simulink model "sampleModel9_EMI_Var"  (R2017a)
settings: Solver=VariableStepAuto  StartTime=0.0  StopTime=10.0  RelTol=1e-3
undefined symbols (not defined in the file or in its folder): DiscIntNeverNeededParam
libraries: simulink x42
settings Model: Creator=cyfuzz  LastModifiedBy=cyfuzz

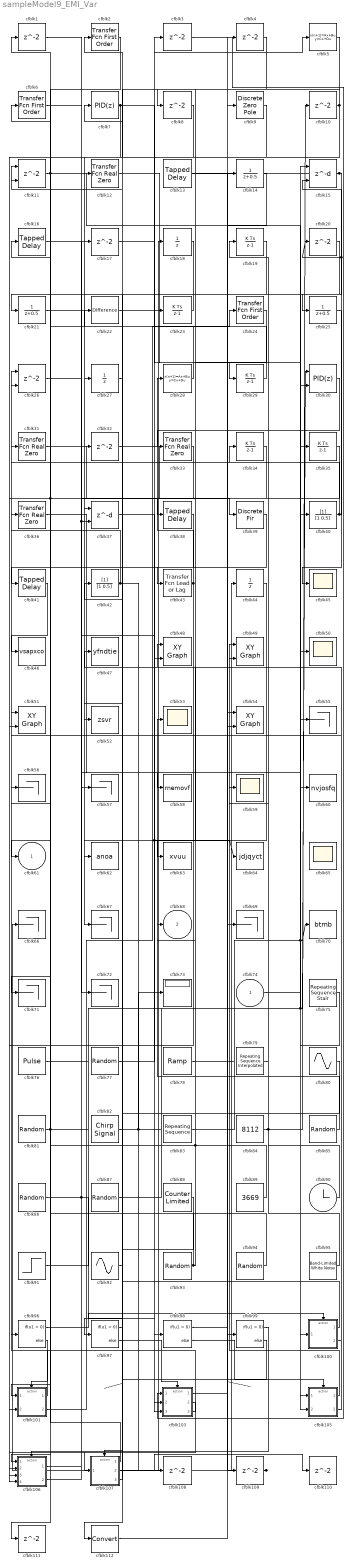
== system sampleModel9_EMI_Var ==
  cfblk74 : Inport
  cfblk{1,3..4,8,10,17,20,32,108..111} (12 alike) : Delay  SampleTime=1
  cfblk100 : Subsystem  TreatAsAtomicUnit=on
  cfblk101 : Subsystem  TreatAsAtomicUnit=on
  cfblk103 : Subsystem  TreatAsAtomicUnit=on
  cfblk105 : Subsystem  TreatAsAtomicUnit=on
  cfblk106 : Subsystem  TreatAsAtomicUnit=on
  cfblk107 : Subsystem  TreatAsAtomicUnit=on
  cfblk11 : Delay  ShowEnablePort=on  SampleTime=1
      settings: InputPortMap=u0,e6
  cfblk112 : DataTypeConversion
  cfblk{12,31,33,36} (4 alike) : simulink/Discrete/Transfer Fcn Real Zero  ZeroZ=0.75  ICPrevInput=0.0  DoSatur=off
      settings: SourceProductName=Simulink  SourceProductBaseCode=SL
  cfblk{13,16,38,41} (4 alike) : simulink/Discrete/Tapped Delay  vinit=0.0  samptime=-1  NumDelays=1  DelayOrder=Oldest  includeCurrent=off
  cfblk14 : DiscreteTransferFcn  SampleTime=1
  cfblk15 : Delay  DelayLengthSource=Input port  SampleTime=1
      settings: InputPortMap=u0,p1
  cfblk18 : UnitDelay
  cfblk{19,23,29,34..35} (5 alike) : DiscreteIntegrator  InitialConditionSetting=State (most efficient)  ICPrevOutput=DiscIntNeverNeededParam  ICPrevScaledInput=DiscIntNeverNeededParam
  cfblk2 : simulink/Discrete/Transfer Fcn First Order  PoleZ=0.95  ICPrevOutput=0.0  DoSatur=off
      settings: SourceProductName=Simulink
  cfblk21 : DiscreteTransferFcn  SampleTime=1
  cfblk22 : simulink/Discrete/Difference  ICPrevInput=0.0  OutMin=[]  OutMax=[]  OutDataTypeStr=Inherit: Inherit via back propagation  OutDataType=fixdt(1, 16)  OutScaling=2^-10  DoSatur=off
  cfblk24 : simulink/Discrete/Transfer Fcn First Order  PoleZ=0.95  ICPrevOutput=0.0  DoSatur=off
      settings: SourceProductName=Simulink
  cfblk25 : DiscreteTransferFcn  SampleTime=1
  cfblk26 : Delay  ShowEnablePort=on  SampleTime=1
      settings: InputPortMap=u0,e6
  cfblk27 : UnitDelay
  cfblk28 : DiscreteStateSpace
  cfblk30 : simulink/Continuous/PID Controller (2DOF)  Controller=PID  TimeDomain=Discrete-time  SampleTime=1  IntegratorMethod=Forward Euler  FilterMethod=Forward Euler  Form=Parallel  UseFilter=on  ControllerParametersSource=internal  P=1  I=1  D=0  N=100  b=1  c=1  InitialConditionSource=internal  InitialConditionForIntegrator=0  InitialConditionForFilter=0  ExternalReset=none  LimitOutput=off  UpperSaturationLimit=inf  LowerSaturationLimit=-inf  LinearizeAsGain=off  AntiWindupMode=none  Kb=1  TrackingMode=off  Kt=1  PParamMin=[]  PParamMax=[]  IParamMin=[]  IParamMax=[]  DParamMin=[]  DParamMax=[]  NParamMin=[]  NParamMax=[]  bParamMin=[]  bParamMax=[]  cParamMin=[]  cParamMax=[]  KbParamMin=[]  KbParamMax=[]  KtParamMin=[]  KtParamMax=[]  POutMin=[]  POutMax=[]  IOutMin=[]  IOutMax=[]  DOutMin=[]  DOutMax=[]  NOutMin=[]  NOutMax=[]  bOutMin=[]  bOutMax=[]  cOutMin=[]  cOutMax=[]  KbOutMin=[]  KbOutMax=[]  KtOutMin=[]  KtOutMax=[]  IntegratorOutMin=[]  IntegratorOutMax=[]  FilterOutMin=[]  FilterOutMax=[]  SumOutMin=[]  SumOutMax=[]  Sum1OutMin=[]  Sum1OutMax=[]  Sum2OutMin=[]  Sum2OutMax=[]  Sum3OutMin=[]  Sum3OutMax=[]  SumI1OutMin=[]  SumI1OutMax=[]  SumI2OutMin=[]  SumI2OutMax=[]  SumI3OutMin=[]  SumI3OutMax=[]  SumDOutMin=[]  SumDOutMax=[]  SaturationOutMin=[]  SaturationOutMax=[]  IntegratorContinuousStateAttributes=''  IntegratorStateMustResolveToSignalObject=off  IntegratorRTWStateStorageClass=Auto  FilterContinuousStateAttributes=''  FilterStateMustResolveToSignalObject=off  FilterRTWStateStorageClass=Auto  DifferentiatorICPrevScaledInput=0  DifferentiatorOutMin=[]  DifferentiatorOutMax=[]  InitialConditionSetting=State (most efficient)
  cfblk37 : Delay  DelayLengthSource=Input port  SampleTime=1
      settings: InputPortMap=u0,p1
  cfblk39 : DiscreteFir  SampleTime=1
  cfblk40 : DiscreteFilter  SampleTime=1
  cfblk42 : DiscreteFilter  SampleTime=1
  cfblk43 : simulink/Discrete/Transfer Fcn Lead or Lag  PoleZ=0.95  ZeroZ=0.75  ICPrevOutput=0.0  ICPrevInput=0.0  DoSatur=off
      settings: SourceProductName=Simulink  SourceProductBaseCode=SL
  cfblk44 : UnitDelay
  cfblk{45,50,53,59,65} (5 alike) : Scope
      cfblk65 settings: Floating=on
  cfblk46 : ToWorkspace  VariableName=vsapxco  SaveFormat=Timeseries  SampleTime=-1
  cfblk47 : ToWorkspace  VariableName=yfndtie  SaveFormat=Timeseries  SampleTime=-1
  cfblk{48..49,51,54} (4 alike) : simulink/Sinks/XY Graph  xmin=-1  xmax=1  ymin=-1  ymax=1  st=-1
  cfblk5 : DiscreteStateSpace
  cfblk52 : ToFile  Filename=zsvr  SaveFormat=Timeseries
  cfblk{55..57,66..67,69,71..72} (8 alike) : Terminator
  cfblk58 : ToWorkspace  VariableName=rnemovf  SaveFormat=Timeseries  SampleTime=-1
  cfblk6 : simulink/Discrete/Transfer Fcn First Order  PoleZ=0.95  ICPrevOutput=0.0  DoSatur=off
      settings: SourceProductName=Simulink
  cfblk60 : ToWorkspace  VariableName=nvjosfq  SaveFormat=Timeseries  SampleTime=-1
  cfblk62 : ToFile  Filename=anoa  SaveFormat=Timeseries
  cfblk63 : ToFile  Filename=xvuu  SaveFormat=Timeseries
  cfblk64 : ToWorkspace  VariableName=jdjqyct  SaveFormat=Timeseries  SampleTime=-1
  cfblk7 : simulink/Continuous/PID Controller  Controller=PID  TimeDomain=Discrete-time  SampleTime=1  IntegratorMethod=Forward Euler  FilterMethod=Forward Euler  Form=Parallel  UseFilter=on  ControllerParametersSource=internal  P=1  I=1  D=0  N=100  InitialConditionSource=internal  InitialConditionForIntegrator=0  InitialConditionForFilter=0  ExternalReset=none  LimitOutput=off  UpperSaturationLimit=inf  LowerSaturationLimit=-inf  LinearizeAsGain=off  AntiWindupMode=none  Kb=1  TrackingMode=off  Kt=1  PParamMin=[]  PParamMax=[]  IParamMin=[]  IParamMax=[]  DParamMin=[]  DParamMax=[]  NParamMin=[]  NParamMax=[]  KbParamMin=[]  KbParamMax=[]  KtParamMin=[]  KtParamMax=[]  POutMin=[]  POutMax=[]  IOutMin=[]  IOutMax=[]  DOutMin=[]  DOutMax=[]  NOutMin=[]  NOutMax=[]  KbOutMin=[]  KbOutMax=[]  KtOutMin=[]  KtOutMax=[]  IntegratorOutMin=[]  IntegratorOutMax=[]  FilterOutMin=[]  FilterOutMax=[]  SumOutMin=[]  SumOutMax=[]  SumI1OutMin=[]  SumI1OutMax=[]  SumI2OutMin=[]  SumI2OutMax=[]  SumI3OutMin=[]  SumI3OutMax=[]  SumDOutMin=[]  SumDOutMax=[]  SaturationOutMin=[]  SaturationOutMax=[]  IntegratorContinuousStateAttributes=''  IntegratorStateMustResolveToSignalObject=off  IntegratorRTWStateStorageClass=Auto  FilterContinuousStateAttributes=''  FilterStateMustResolveToSignalObject=off  FilterRTWStateStorageClass=Auto  DifferentiatorICPrevScaledInput=0  DifferentiatorOutMin=[]  DifferentiatorOutMax=[]  InitialConditionSetting=State (most efficient)
  cfblk70 : ToFile  Filename=btmb  SaveFormat=Timeseries
  cfblk73 : Display
  cfblk75 : simulink/Sources/Repeating Sequence Stair  OutValues=[3 1 4 2 1].'  tsamp=-1  OutMin=[]  OutMax=[]  OutDataTypeStr=double  OutputDataTypeScalingMode=double  OutDataType=fixdt(0,8)  ConRadixGroup=Best Precision: Vector-wise  OutScaling=2^-12
  cfblk76 : DiscretePulseGenerator  PulseType=Time based  Period=10  PulseWidth=5
  cfblk{77,81,85..87,93..94} (7 alike) : RandomNumber  SampleTime=0.1
  cfblk78 : simulink/Sources/Ramp  slope=1  start=0  X0=0
  cfblk79 : simulink/Sources/Repeating Sequence Interpolated  OutValues=[3 1 4 2 1].'  TimeValues=[0 0.1 0.5 0.6 1].'  LookUpMeth=Interpolation-Use End Values  tsamp=0.01  OutMin=[]  OutMax=[]  OutDataTypeStr=double  OutputDataTypeScalingMode=double  OutDataType=fixdt(0,8)  OutScaling=2^-10
  cfblk80 : Sin  SampleTime=0
  cfblk82 : simulink/Sources/Chirp Signal  f1=0.1  T=100  f2=1
  cfblk83 : simulink/Sources/Repeating Sequence  rep_seq_t=[0 2]  rep_seq_y=[0 2]
  cfblk84 : Constant  Value=8112
  cfblk88 : simulink/Sources/Counter Limited  uplimit=7  tsamp=-1
  cfblk89 : Constant  Value=3669
  cfblk9 : DiscreteZeroPole  Poles=[0 0.5]  Gain=1
  cfblk90 : Clock
  cfblk91 : Step  After=97  SampleTime=0
  cfblk92 : Sin  SampleTime=0
  cfblk95 : simulink/Sources/Band-Limited White Noise  Cov=[0.1]  Ts=0.1  seed=[23341]
  cfblk{96..99} (4 alike) : If  SampleTime=1
  cfblk61 : Outport
  cfblk68 : Outport  Port=2
  wires:
  cfblk85/1 -> cfblk53/1
  cfblk101/1(cfblk2) -> cfblk26/1
  cfblk8/1 -> cfblk67/1
  cfblk101/2(cfblk13) -> cfblk24/1
  cfblk84/1 -> cfblk10/1, cfblk59/1
  cfblk86/1 -> cfblk57/1, cfblk103/3(cfblk7)
  cfblk92/1 -> cfblk2/1
  cfblk9/1 -> cfblk41/1
  cfblk10/1 -> cfblk8/1, cfblk33/1
  cfblk106/1(cfblk2) -> cfblk17/1
  cfblk43/1 -> cfblk28/1, cfblk106/4(cfblk8)
  cfblk20/1 -> cfblk97/1
  cfblk30/1 -> cfblk63/1
  cfblk76/1 -> cfblk30/1, cfblk30/2
  cfblk11/1 -> cfblk35/1, cfblk111/1
  cfblk38/1 -> cfblk106/1(cfblk1)
  cfblk25/1 -> cfblk45/1
  cfblk95/1 -> cfblk19/1
  cfblk40/1 -> cfblk15/2, cfblk20/1, cfblk26/2
  cfblk105/1(cfblk2) -> cfblk49/1
  cfblk21/1 -> cfblk27/1
  cfblk42/1 -> cfblk31/1, cfblk108/1
  cfblk18/1 -> cfblk37/1
  cfblk22/1 -> cfblk60/1
  cfblk36/1 -> cfblk105/1(cfblk1)
  cfblk74/1 -> cfblk40/1
  cfblk91/1 -> cfblk55/1
  cfblk12/1 -> cfblk100/1(cfblk1)
  cfblk27/1 -> cfblk7/1
  cfblk31/1 -> cfblk54/1
  cfblk3/1 -> cfblk103/1(cfblk1)
  cfblk80/1 -> cfblk107/1(cfblk1)
  cfblk14/1 -> cfblk54/2
  cfblk77/1 -> cfblk3/1
  cfblk87/1 -> cfblk4/1
  cfblk23/1 -> cfblk21/1
  cfblk15/1 -> cfblk25/1, cfblk13/1
  cfblk2/1 -> cfblk71/1
  cfblk106/2(cfblk9) -> cfblk32/1
  cfblk7/1 -> cfblk29/1, cfblk101/2(cfblk12)
  cfblk81/1 -> cfblk56/1, cfblk23/1
  cfblk103/1(cfblk2) -> cfblk99/1
  cfblk93/1 -> cfblk6/1, cfblk48/1
  cfblk37/1 -> cfblk98/1, cfblk64/1
  cfblk5/1 -> cfblk12/1
  cfblk94/1 -> cfblk22/1
  cfblk100/1(cfblk2) -> cfblk42/1
  cfblk89/1 -> cfblk16/1, cfblk68/1
  cfblk105/2(cfblk13) -> cfblk51/1
  cfblk4/1 -> cfblk43/1
  cfblk75/1 -> cfblk105/2(cfblk12)
  cfblk41/1 -> cfblk46/1
  cfblk24/1 -> cfblk38/1
  cfblk17/1 -> cfblk5/1
  cfblk79/1 -> cfblk49/2
  cfblk100/2(cfblk10) -> cfblk47/1
  cfblk16/1 -> cfblk72/1
  cfblk78/1 -> cfblk15/1
  cfblk6/1 -> cfblk39/1
  cfblk44/1 -> cfblk62/1
  cfblk39/1 -> cfblk103/2(cfblk6)
  cfblk35/1 -> cfblk52/1
  cfblk34/1 -> cfblk106/2(cfblk6)
  cfblk107/1(cfblk2) -> cfblk36/1
  cfblk103/2(cfblk8) -> cfblk106/3(cfblk7)
  cfblk83/1 -> cfblk70/1, cfblk50/1
  cfblk32/1 -> cfblk69/1
  cfblk26/1 -> cfblk37/2, cfblk48/2
  cfblk19/1 -> cfblk101/1(cfblk1)
  cfblk28/1 -> cfblk11/1
  cfblk1/1 -> cfblk58/1
  cfblk29/1 -> cfblk1/1
  cfblk33/1 -> cfblk61/1, cfblk51/2
  cfblk82/1 -> cfblk14/1, cfblk73/1
  cfblk90/1 -> cfblk34/1
  cfblk103/3(cfblk9) -> cfblk96/1
  cfblk107/3(cfblk7) -> cfblk11/2
  cfblk96/1 -> cfblk100/Action
  cfblk96/2 -> cfblk101/Action
  cfblk97/1 -> ?
  cfblk97/2 -> cfblk103/Action
  cfblk98/1 -> ?
  cfblk98/2 -> cfblk105/Action
  cfblk99/1 -> cfblk106/Action
  cfblk99/2 -> cfblk107/Action
  cfblk13/1 -> cfblk109/1
  cfblk107/2(cfblk6) -> cfblk110/1
  cfblk88/1 -> cfblk112/1
  cfblk112/1 -> cfblk9/1
  cfblk109/1 -> cfblk18/1, cfblk44/1, cfblk66/1

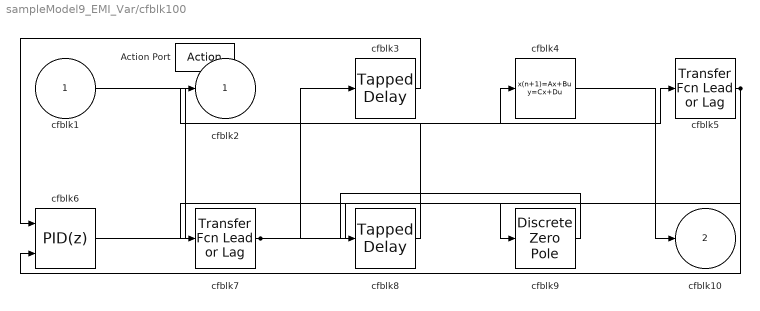
== system sampleModel9_EMI_Var/cfblk100 ==
  cfblk1 : Inport
  Action Port : ActionPort  ActionType=then
  cfblk3 : simulink/Discrete/Tapped Delay  vinit=0.0  samptime=-1  NumDelays=1  DelayOrder=Oldest  includeCurrent=off
  cfblk4 : DiscreteStateSpace  SampleTime=-1
  cfblk5 : simulink/Discrete/Transfer Fcn Lead or Lag  PoleZ=0.95  ZeroZ=0.75  ICPrevOutput=0.0  ICPrevInput=0.0  DoSatur=off
      settings: SourceProductName=Simulink  SourceProductBaseCode=SL
  cfblk6 : simulink/Continuous/PID Controller (2DOF)  Controller=PID  TimeDomain=Discrete-time  SampleTime=-1  IntegratorMethod=Forward Euler  FilterMethod=Forward Euler  Form=Parallel  UseFilter=on  ControllerParametersSource=internal  P=1  I=1  D=0  N=100  b=1  c=1  InitialConditionSource=internal  InitialConditionForIntegrator=0  InitialConditionForFilter=0  ExternalReset=none  LimitOutput=off  UpperSaturationLimit=inf  LowerSaturationLimit=-inf  LinearizeAsGain=off  AntiWindupMode=none  Kb=1  TrackingMode=off  Kt=1  PParamMin=[]  PParamMax=[]  IParamMin=[]  IParamMax=[]  DParamMin=[]  DParamMax=[]  NParamMin=[]  NParamMax=[]  bParamMin=[]  bParamMax=[]  cParamMin=[]  cParamMax=[]  KbParamMin=[]  KbParamMax=[]  KtParamMin=[]  KtParamMax=[]  POutMin=[]  POutMax=[]  IOutMin=[]  IOutMax=[]  DOutMin=[]  DOutMax=[]  NOutMin=[]  NOutMax=[]  bOutMin=[]  bOutMax=[]  cOutMin=[]  cOutMax=[]  KbOutMin=[]  KbOutMax=[]  KtOutMin=[]  KtOutMax=[]  IntegratorOutMin=[]  IntegratorOutMax=[]  FilterOutMin=[]  FilterOutMax=[]  SumOutMin=[]  SumOutMax=[]  Sum1OutMin=[]  Sum1OutMax=[]  Sum2OutMin=[]  Sum2OutMax=[]  Sum3OutMin=[]  Sum3OutMax=[]  SumI1OutMin=[]  SumI1OutMax=[]  SumI2OutMin=[]  SumI2OutMax=[]  SumI3OutMin=[]  SumI3OutMax=[]  SumDOutMin=[]  SumDOutMax=[]  SaturationOutMin=[]  SaturationOutMax=[]  IntegratorContinuousStateAttributes=''  IntegratorStateMustResolveToSignalObject=off  IntegratorRTWStateStorageClass=Auto  FilterContinuousStateAttributes=''  FilterStateMustResolveToSignalObject=off  FilterRTWStateStorageClass=Auto  DifferentiatorICPrevScaledInput=0  DifferentiatorOutMin=[]  DifferentiatorOutMax=[]  InitialConditionSetting=State (most efficient)
  cfblk7 : simulink/Discrete/Transfer Fcn Lead or Lag  PoleZ=0.95  ZeroZ=0.75  ICPrevOutput=0.0  ICPrevInput=0.0  DoSatur=off
      settings: SourceProductName=Simulink  SourceProductBaseCode=SL
  cfblk8 : simulink/Discrete/Tapped Delay  vinit=0.0  samptime=-1  NumDelays=1  DelayOrder=Oldest  includeCurrent=off
  cfblk9 : DiscreteZeroPole  Poles=[0 0.5]  Gain=1  SampleTime=-1
  cfblk2 : Outport
  cfblk10 : Outport  Port=2
  wires:
  cfblk1/1 -> cfblk5/1
  cfblk6/1 -> cfblk4/1
  cfblk3/1 -> cfblk6/1
  cfblk5/1 -> cfblk6/2, cfblk7/1
  cfblk7/1 -> cfblk9/1, cfblk3/1
  cfblk4/1 -> cfblk10/1
  cfblk9/1 -> cfblk8/1
  cfblk8/1 -> cfblk2/1

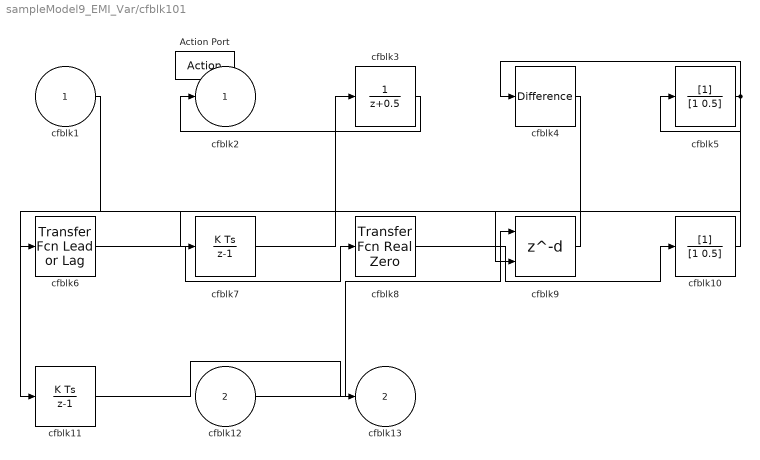
== system sampleModel9_EMI_Var/cfblk101 ==
  cfblk1 : Inport
  cfblk12 : Inport  Port=2
  Action Port : ActionPort  ActionType=else
  cfblk10 : DiscreteFilter
  cfblk11 : DiscreteIntegrator  InitialConditionSetting=State (most efficient)  SampleTime=-1  ICPrevOutput=DiscIntNeverNeededParam  ICPrevScaledInput=DiscIntNeverNeededParam
  cfblk3 : DiscreteTransferFcn
  cfblk4 : simulink/Discrete/Difference  ICPrevInput=0.0  OutMin=[]  OutMax=[]  OutDataTypeStr=Inherit: Inherit via back propagation  OutDataType=fixdt(1, 16)  OutScaling=2^-10  DoSatur=off
  cfblk5 : DiscreteFilter
  cfblk6 : simulink/Discrete/Transfer Fcn Lead or Lag  PoleZ=0.95  ZeroZ=0.75  ICPrevOutput=0.0  ICPrevInput=0.0  DoSatur=off
      settings: SourceProductName=Simulink  SourceProductBaseCode=SL
  cfblk7 : DiscreteIntegrator  InitialConditionSetting=State (most efficient)  SampleTime=-1  ICPrevOutput=DiscIntNeverNeededParam  ICPrevScaledInput=DiscIntNeverNeededParam
  cfblk8 : simulink/Discrete/Transfer Fcn Real Zero  ZeroZ=0.75  ICPrevInput=0.0  DoSatur=off
      settings: SourceProductName=Simulink  SourceProductBaseCode=SL
  cfblk9 : Delay  DelayLengthSource=Input port
      settings: InputPortMap=u0,p1
  cfblk2 : Outport
  cfblk13 : Outport  Port=2
  wires:
  cfblk4/1 -> cfblk11/1
  cfblk8/1 -> cfblk10/1
  cfblk6/1 -> cfblk8/1
  cfblk3/1 -> cfblk2/1
  cfblk1/1 -> cfblk6/1
  cfblk9/1 -> cfblk7/1
  cfblk12/1 -> cfblk9/1
  cfblk7/1 -> cfblk3/1
  cfblk10/1 -> cfblk5/1
  cfblk5/1 -> cfblk4/1, cfblk9/2
  cfblk11/1 -> cfblk13/1

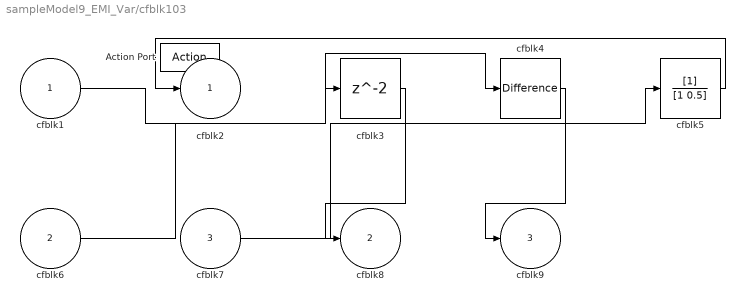
== system sampleModel9_EMI_Var/cfblk103 ==
  cfblk1 : Inport
  cfblk6 : Inport  Port=2
  cfblk7 : Inport  Port=3
  Action Port : ActionPort  ActionType=else
  cfblk3 : Delay
  cfblk4 : simulink/Discrete/Difference  ICPrevInput=0.0  OutMin=[]  OutMax=[]  OutDataTypeStr=Inherit: Inherit via back propagation  OutDataType=fixdt(1, 16)  OutScaling=2^-10  DoSatur=off
  cfblk5 : DiscreteFilter
  cfblk2 : Outport
  cfblk8 : Outport  Port=2
  cfblk9 : Outport  Port=3
  wires:
  cfblk7/1 -> cfblk5/1
  cfblk5/1 -> cfblk2/1
  cfblk1/1 -> cfblk4/1
  cfblk4/1 -> cfblk9/1
  cfblk6/1 -> cfblk3/1
  cfblk3/1 -> cfblk8/1

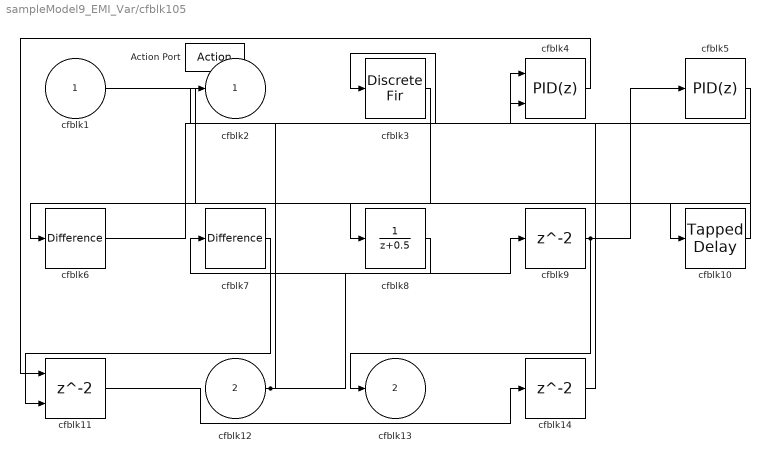
== system sampleModel9_EMI_Var/cfblk105 ==
  cfblk1 : Inport
  cfblk12 : Inport  Port=2
  Action Port : ActionPort  ActionType=else
  cfblk10 : simulink/Discrete/Tapped Delay  vinit=0.0  samptime=-1  NumDelays=1  DelayOrder=Oldest  includeCurrent=off
  cfblk11 : Delay  ShowEnablePort=on
      settings: InputPortMap=u0,e6
  cfblk14 : Delay
  cfblk3 : DiscreteFir
  cfblk4 : simulink/Continuous/PID Controller (2DOF)  Controller=PID  TimeDomain=Discrete-time  SampleTime=-1  IntegratorMethod=Forward Euler  FilterMethod=Forward Euler  Form=Parallel  UseFilter=on  ControllerParametersSource=internal  P=1  I=1  D=0  N=100  b=1  c=1  InitialConditionSource=internal  InitialConditionForIntegrator=0  InitialConditionForFilter=0  ExternalReset=none  LimitOutput=off  UpperSaturationLimit=inf  LowerSaturationLimit=-inf  LinearizeAsGain=off  AntiWindupMode=none  Kb=1  TrackingMode=off  Kt=1  PParamMin=[]  PParamMax=[]  IParamMin=[]  IParamMax=[]  DParamMin=[]  DParamMax=[]  NParamMin=[]  NParamMax=[]  bParamMin=[]  bParamMax=[]  cParamMin=[]  cParamMax=[]  KbParamMin=[]  KbParamMax=[]  KtParamMin=[]  KtParamMax=[]  POutMin=[]  POutMax=[]  IOutMin=[]  IOutMax=[]  DOutMin=[]  DOutMax=[]  NOutMin=[]  NOutMax=[]  bOutMin=[]  bOutMax=[]  cOutMin=[]  cOutMax=[]  KbOutMin=[]  KbOutMax=[]  KtOutMin=[]  KtOutMax=[]  IntegratorOutMin=[]  IntegratorOutMax=[]  FilterOutMin=[]  FilterOutMax=[]  SumOutMin=[]  SumOutMax=[]  Sum1OutMin=[]  Sum1OutMax=[]  Sum2OutMin=[]  Sum2OutMax=[]  Sum3OutMin=[]  Sum3OutMax=[]  SumI1OutMin=[]  SumI1OutMax=[]  SumI2OutMin=[]  SumI2OutMax=[]  SumI3OutMin=[]  SumI3OutMax=[]  SumDOutMin=[]  SumDOutMax=[]  SaturationOutMin=[]  SaturationOutMax=[]  IntegratorContinuousStateAttributes=''  IntegratorStateMustResolveToSignalObject=off  IntegratorRTWStateStorageClass=Auto  FilterContinuousStateAttributes=''  FilterStateMustResolveToSignalObject=off  FilterRTWStateStorageClass=Auto  DifferentiatorICPrevScaledInput=0  DifferentiatorOutMin=[]  DifferentiatorOutMax=[]  InitialConditionSetting=State (most efficient)
  cfblk5 : simulink/Continuous/PID Controller  Controller=PID  TimeDomain=Discrete-time  SampleTime=-1  IntegratorMethod=Forward Euler  FilterMethod=Forward Euler  Form=Parallel  UseFilter=on  ControllerParametersSource=internal  P=1  I=1  D=0  N=100  InitialConditionSource=internal  InitialConditionForIntegrator=0  InitialConditionForFilter=0  ExternalReset=none  LimitOutput=off  UpperSaturationLimit=inf  LowerSaturationLimit=-inf  LinearizeAsGain=off  AntiWindupMode=none  Kb=1  TrackingMode=off  Kt=1  PParamMin=[]  PParamMax=[]  IParamMin=[]  IParamMax=[]  DParamMin=[]  DParamMax=[]  NParamMin=[]  NParamMax=[]  KbParamMin=[]  KbParamMax=[]  KtParamMin=[]  KtParamMax=[]  POutMin=[]  POutMax=[]  IOutMin=[]  IOutMax=[]  DOutMin=[]  DOutMax=[]  NOutMin=[]  NOutMax=[]  KbOutMin=[]  KbOutMax=[]  KtOutMin=[]  KtOutMax=[]  IntegratorOutMin=[]  IntegratorOutMax=[]  FilterOutMin=[]  FilterOutMax=[]  SumOutMin=[]  SumOutMax=[]  SumI1OutMin=[]  SumI1OutMax=[]  SumI2OutMin=[]  SumI2OutMax=[]  SumI3OutMin=[]  SumI3OutMax=[]  SumDOutMin=[]  SumDOutMax=[]  SaturationOutMin=[]  SaturationOutMax=[]  IntegratorContinuousStateAttributes=''  IntegratorStateMustResolveToSignalObject=off  IntegratorRTWStateStorageClass=Auto  FilterContinuousStateAttributes=''  FilterStateMustResolveToSignalObject=off  FilterRTWStateStorageClass=Auto  DifferentiatorICPrevScaledInput=0  DifferentiatorOutMin=[]  DifferentiatorOutMax=[]  InitialConditionSetting=State (most efficient)
  cfblk6 : simulink/Discrete/Difference  ICPrevInput=0.0  OutMin=[]  OutMax=[]  OutDataTypeStr=Inherit: Inherit via back propagation  OutDataType=fixdt(1, 16)  OutScaling=2^-10  DoSatur=off
  cfblk7 : simulink/Discrete/Difference  ICPrevInput=0.0  OutMin=[]  OutMax=[]  OutDataTypeStr=Inherit: Inherit via back propagation  OutDataType=fixdt(1, 16)  OutScaling=2^-10  DoSatur=off
  cfblk8 : DiscreteTransferFcn
  cfblk9 : Delay
  cfblk2 : Outport
  cfblk13 : Outport  Port=2
  wires:
  cfblk3/1 -> cfblk6/1
  cfblk10/1 -> cfblk3/1
  cfblk1/1 -> cfblk10/1
  cfblk8/1 -> cfblk7/1
  cfblk4/1 -> cfblk11/1
  cfblk5/1 -> cfblk8/1
  cfblk7/1 -> cfblk11/2
  cfblk6/1 -> cfblk4/1
  cfblk12/1 -> cfblk2/1, cfblk9/1
  cfblk9/1 -> cfblk13/1, cfblk5/1
  cfblk11/1 -> cfblk14/1
  cfblk14/1 -> cfblk4/2

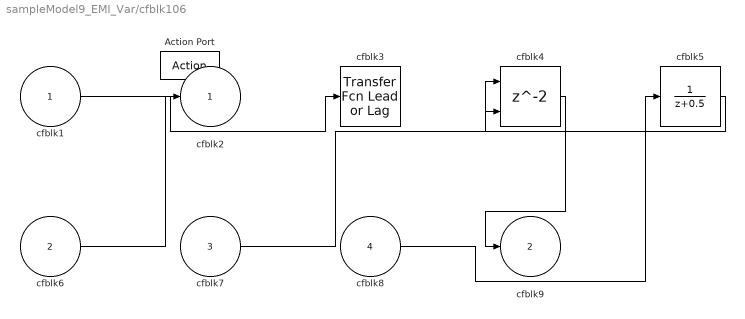
== system sampleModel9_EMI_Var/cfblk106 ==
  cfblk1 : Inport
  cfblk6 : Inport  Port=2
  cfblk7 : Inport  Port=3
  cfblk8 : Inport  Port=4
  Action Port : ActionPort  ActionType=then
  cfblk3 : simulink/Discrete/Transfer Fcn Lead or Lag  PoleZ=0.95  ZeroZ=0.75  ICPrevOutput=0.0  ICPrevInput=0.0  DoSatur=off
      settings: SourceProductName=Simulink  SourceProductBaseCode=SL
  cfblk4 : Delay  ShowEnablePort=on
      settings: InputPortMap=u0,e6
  cfblk5 : DiscreteTransferFcn
  cfblk2 : Outport
  cfblk9 : Outport  Port=2
  wires:
  cfblk4/1 -> cfblk9/1
  cfblk1/1 -> cfblk3/1
  cfblk6/1 -> cfblk2/1
  cfblk7/1 -> cfblk4/1
  cfblk8/1 -> cfblk5/1
  cfblk5/1 -> cfblk4/2

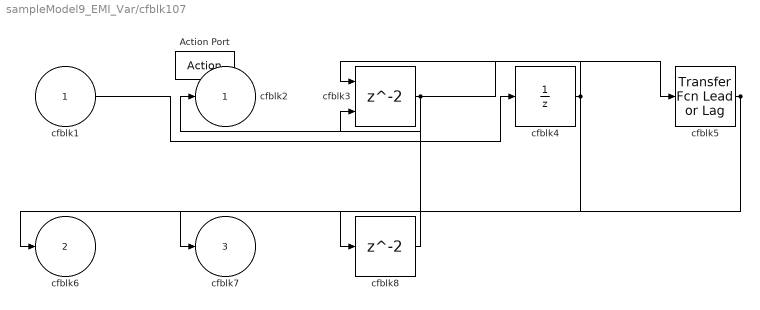
== system sampleModel9_EMI_Var/cfblk107 ==
  cfblk1 : Inport
  Action Port : ActionPort  ActionType=else
  cfblk3 : Delay  ShowEnablePort=on
      settings: InputPortMap=u0,e6
  cfblk4 : UnitDelay  SampleTime=-1
  cfblk5 : simulink/Discrete/Transfer Fcn Lead or Lag  PoleZ=0.95  ZeroZ=0.75  ICPrevOutput=0.0  ICPrevInput=0.0  DoSatur=off
      settings: SourceProductName=Simulink  SourceProductBaseCode=SL
  cfblk8 : Delay
  cfblk2 : Outport
  cfblk6 : Outport  Port=2
  cfblk7 : Outport  Port=3
  wires:
  cfblk3/1 -> cfblk2/1, cfblk5/1
  cfblk5/1 -> cfblk7/1, cfblk8/1
  cfblk1/1 -> cfblk4/1
  cfblk4/1 -> cfblk3/1, cfblk6/1
  cfblk8/1 -> cfblk3/2
